simulink model "test"  (R2023a)
settings: Solver=FixedStepAuto  StartTime=0.0  StopTime=25  RelTol=1e-3
libraries: simulink x3
settings Model: Creator=19856  LastModifiedBy=19856
settings ModelReferenceCC: ModelReferenceNumInstancesAllowed=Single

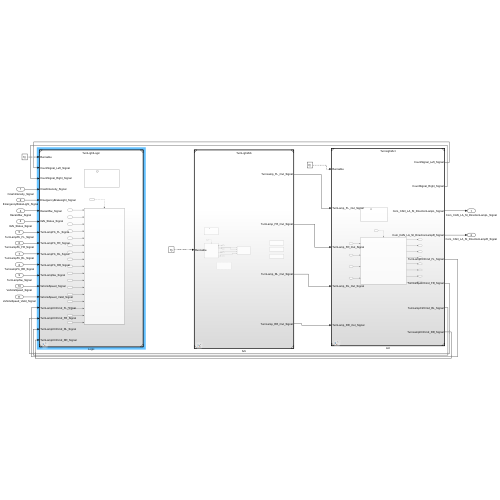
[thumbnail: Simulink's stored preview of the top-level diagram]
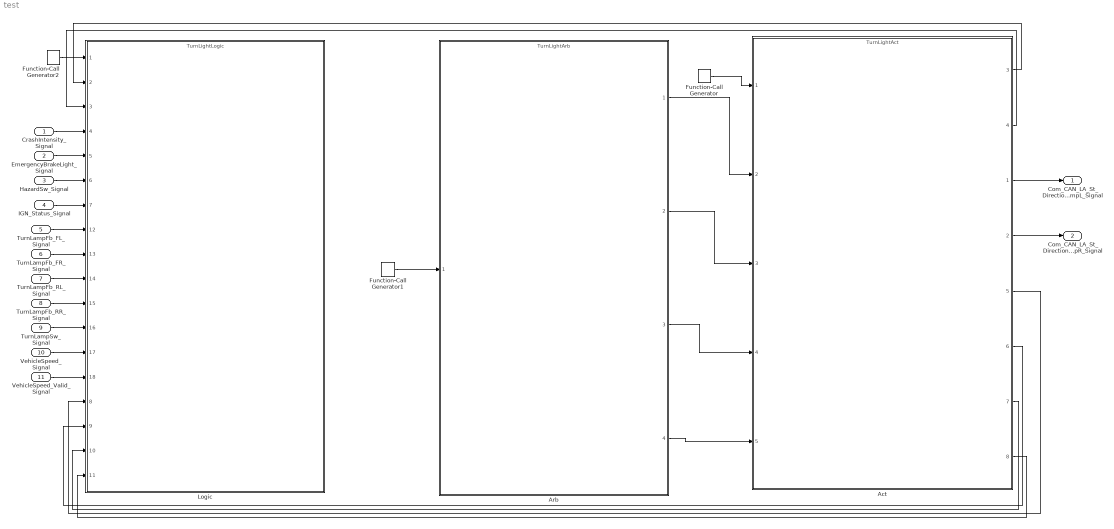
== system test ==
  CrashIntensity_Signal : Inport
  EmergencyBrakeLight_Signal : Inport  Port=2
  HazardSw_Signal : Inport  Port=3
  IGN_Status_Signal : Inport  Port=4
  TurnLampFb_FL_Signal : Inport  Port=5
  TurnLampFb_FR_Signal : Inport  Port=6
  TurnLampFb_RL_Signal : Inport  Port=7
  TurnLampFb_RR_Signal : Inport  Port=8
  TurnLampSw_Signal : Inport  Port=9
  VehicleSpeed_Signal : Inport  Port=10
  VehicleSpeed_Valid_Signal : Inport  Port=11
  Act : ModelReference  ModelNameDialog=TurnLightAct.slx  SimulationMode=Normal  ScheduleRates=on  ModelReferenceVersion=1.4
      settings: PortSchema="{\"entries\":[{\"content\":{\"sides\":[{\"content\":{\"connectorIds\":[\"In1\",\"In2\",\"In3\",\"In4\",\"In5\"]},\"type\":\"ConnectorPlacement.EquallySpacedRectSide\",\"uuid\":\"9db016ed-8d5d-46b2-8cf3-1596fa1533ac\"},{\"content\":{\"connectorIds\":[\"Out3\",\"Out4\",\"Out1\",\"Out2\",\"Out5\",\"Out6\",\"Out7\",\"Out8\"],\"side\":\"RIGHT\"},\"type\":\"ConnectorPlacement.EquallySpacedRectSide\",\"uuid\":\"66bd8779-7145-4141-af81-846e3f86f0c5\"},{\"content\":{\"side\":\"TOP\"},\"type\":\"ConnectorPlacement.EquallySpacedRectSide\",\"uuid\":\"fe872fd0-8f6e-4fa7-bc5f-bcc6fe3f2101\"}]},\"type\":\"ConnectorPlacement.EquallySpacedConnector\",\"uuid\":\"c8caacec-79c2-45bf-84d0-69947bad4877\"}],\"packageUris\":[\"http://schema.mathworks.com/mf0/Connector/R2020b\"],\"version\":\"1.0\"}"
  Arb : ModelReference  ModelNameDialog=TurnLightArb.slx  SimulationMode=Normal  ScheduleRates=on  ModelReferenceVersion=1.8
  Function-Call Generator : simulink/Ports & Subsystems/Function-Call Generator  sample_time=0.01  numberOfIterations=1  DisallowWideOutput=off
  Function-Call Generator1 : simulink/Ports & Subsystems/Function-Call Generator  sample_time=0.01  numberOfIterations=1  DisallowWideOutput=off
  Function-Call Generator2 : simulink/Ports & Subsystems/Function-Call Generator  sample_time=0.01  numberOfIterations=1  DisallowWideOutput=off
  Logic : ModelReference  ModelNameDialog=TurnLightLogic.slx  SimulationMode=Normal  ScheduleRates=on  ModelReferenceVersion=1.15
      settings: PortSchema="{\"entries\":[{\"content\":{\"sides\":[{\"content\":{\"connectorIds\":[\"In1\",\"In2\",\"In3\",\"In4\",\"In5\",\"In6\",\"In7\",\"In12\",\"In13\",\"In14\",\"In15\",\"In16\",\"In17\",\"In18\",\"In8\",\"In9\",\"In10\",\"In11\"]},\"type\":\"ConnectorPlacement.EquallySpacedRectSide\",\"uuid\":\"53959260-4ac4-4cfa-90df-7ebdf580062d\"},{\"content\":{\"side\":\"RIGHT\"},\"type\":\"ConnectorPlacement.EquallySpacedRectSide\",\"uuid\":\"c4578714-1ded-481b-a9e9-f765b9e7f973\"},{\"content\":{\"side\":\"TOP\"},\"type\":\"ConnectorPlacement.EquallySpacedRectSide\",\"uuid\":\"b603b901-896c-45d2-80e3-6d8cbb6265dc\"}]},\"type\":\"ConnectorPlacement.EquallySpacedConnector\",\"uuid\":\"7a339c31-6632-4df0-a4c0-5078d3c58a16\"}],\"packageUris\":[\"http://schema.mathworks.com/mf0/Connector/R2020b\"],\"version\":\"1.0\"}"
  Com_CAN_LA_St_DirectionLampL_Signal : Outport
  Com_CAN_LA_St_DirectionLampR_Signal : Outport  Port=2
  wires:
  Arb/4 -> Act/5
  Arb/3 -> Act/4
  Arb/2 -> Act/3
  Arb/1 -> Act/2
  Function-Call Generator/1 -> Act/1
  Function-Call Generator1/1 -> Arb/1
  Function-Call Generator2/1 -> Logic/1
  Act/3 -> Logic/2
  Act/4 -> Logic/3
  Act/8 -> Logic/11
  Act/7 -> Logic/10
  Act/6 -> Logic/9
  Act/5 -> Logic/8
  CrashIntensity_Signal/1 -> Logic/4
  EmergencyBrakeLight_Signal/1 -> Logic/5
  HazardSw_Signal/1 -> Logic/6
  IGN_Status_Signal/1 -> Logic/7
  TurnLampFb_FL_Signal/1 -> Logic/12
  TurnLampFb_FR_Signal/1 -> Logic/13
  TurnLampFb_RL_Signal/1 -> Logic/14
  TurnLampFb_RR_Signal/1 -> Logic/15
  TurnLampSw_Signal/1 -> Logic/16
  VehicleSpeed_Signal/1 -> Logic/17
  VehicleSpeed_Valid_Signal/1 -> Logic/18
  Act/1 -> Com_CAN_LA_St_DirectionLampL_Signal/1
  Act/2 -> Com_CAN_LA_St_DirectionLampR_Signal/1
